simulink model "open_loop"  (R2023b)
settings: Solver=VariableStepAuto  StartTime=0.0  StopTime=0.1  RelTol=1e-3
undefined symbols (not defined in the file): a_m, config, K_g, K_m
settings Model: Creator=foderking  LastModifiedBy=foderking

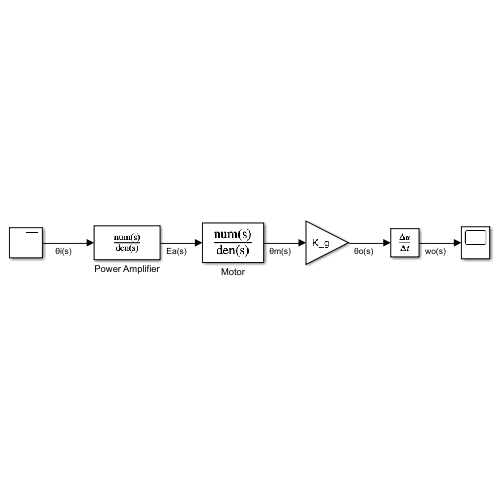
[thumbnail: Simulink's stored preview of the top-level diagram]
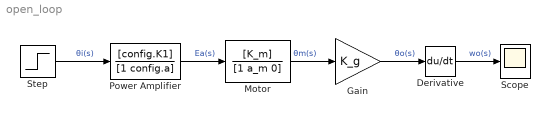
== system open_loop ==
  Derivative : Derivative
  Gain : Gain  Gain=K_g
  Motor : TransferFcn  Numerator=[K_m]  Denominator=[1 a_m 0]
  Power Amplifier : TransferFcn  Numerator=[config.K1]  Denominator=[1 config.a]
  Scope : Scope
  Step : Step  Time=0  SampleTime=0
  wires:
  Step/1 -> Power Amplifier/1  "θi(s)"
  Gain/1 -> Derivative/1  "θo(s)"
  Motor/1 -> Gain/1  "θm(s)"
  Power Amplifier/1 -> Motor/1  "Ea(s)"
  Derivative/1 -> Scope/1  "wo(s)"
